simulink model "Tx_sim"  (R2021b)
settings: Solver=VariableStepAuto  StartTime=0.0  StopTime=10.0  RelTol=1e-3
settings Model: Creator=Blade  LastModifiedBy=Blade

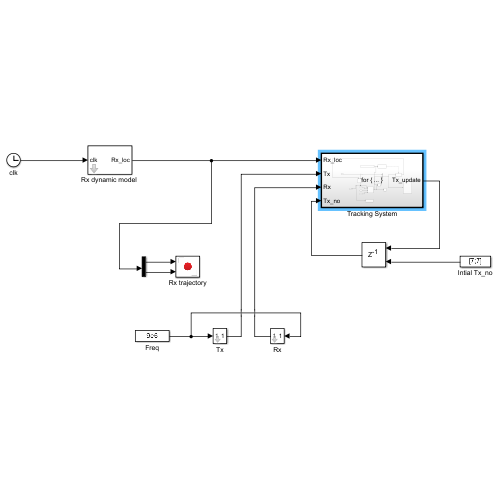
[thumbnail: Simulink's stored preview of the top-level diagram]
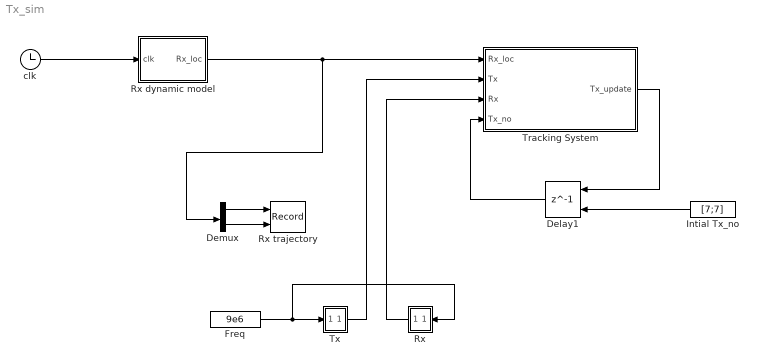
== system Tx_sim ==
  Delay1 : Delay  DelayLength=1  InitialConditionSource=Input port  InitialCondition=[2,2]
      settings: InputPortMap=u0,p4
  Demux : Demux  Outputs=2
  Freq : Constant  Value=9e6
  Intial Tx_no : Constant  Value=[7;7]  VectorParams1D=off
  Rx : Subsystem  mask{dout=1/3*100e-3, phi=0.15, s=800e-6, w=1200e-6, CP=0, SR=0.01}
      mask prompts: dout "out diameter"; phi "fillfact"; s "track spacing"; w "track width"; CP "parasitic capacitance"; SR "source resistance"
      mask TypeOptions dout: Constant1/Value
      mask TypeOptions phi: Constant2/Value
      mask TypeOptions s: Constant3/Value
      mask TypeOptions w: Constant4/Value
      mask TypeOptions CP: Constant6/Value
      mask TypeOptions SR: Constant7/Value
  "Rx dynamic model " : Subsystem  mask{initx=1/2*100e-3*(7+1), inity=1/2*100e-3*(7+1), v_min=[0.01,0.01], v_max=[0.01,0.01]}
      mask prompts: initx "Rx initial x"; inity "Rx initial y"; v_min "Rx min speed"; v_max "Rx max speed"
      mask TypeOptions initx: Delay1/InitialCondition
      mask TypeOptions inity: Delay2/InitialCondition
      mask TypeOptions v_min: Constant/Value
      mask TypeOptions v_max: Constant1/Value
  Rx trajectory : Record  FileSettingsInternal="{\"entries\":[{\"content\":{\"excelSettings\":{\"content\":{},\"type\":\"Streamout.ExcelSettings\"}},\"type\":\"Streamout.FileSettingStorage\",\"uuid\":\"5ea7622f-e3f2-434e-8594-dca06b2b01b1\"}],\"packageUris\":[\"http://schema.mathworks.com/mf0/streamout_blocks/R2020a\"],\"version\":\"1.0\"}"  Layout=[1 1]  SignalsInternal="{\"entries\":[{\"content\":{\"signals\":[{\"content\":{\"blockPath\":[\"untitled/Rx trajectory\"],\"channel\":[],\"dimensions\":[1],\"domain\":\"untitled/Rx trajectory\",\"lineColor\":\"#22b573\",\"plots\":[],\"port\":1,\"sid\":[\"\"],\"signalID\":1150986,\"signalName\":\"Demux:1\"},\"type\":\"RecordBlkView.Signal\",\"uuid\":\"ce63fc5f-71f3-4bbf-96f5-20283097e031\"},{\"content\":{\"blockPath\":[\"untitled/Rx trajectory\"],\"channel\":[],\"dimensions\":[1],\"domain\":\"untitled/Rx trajectory\",\"lineColor\":\"#0072bd\",\"plots\":[],\"port\":2,\"sid\":[\"\"],\"signalID\":1150990,\"signalName\":\"Demux:2\"},\"type\":\"RecordBlkView.Signal\",\"uuid\":\"feeefa71-ac5c-4467-a179-d29ba9ae9525\"}]},\"type\":\"RecordBlkView.InputSignals\",\"uuid\":\"cc4d89dd-a1d8-473b-8fe9-6d08d22a2a17\"}],\"packageUris\":[\"http://schema.mathworks.com/mf0/streamout_blocks/R2020a\"],\"version\":\"1.0\"}"  VisualizationBindings="{\"xyplotplugin\":{\"info\":[{\"series\":[],\"subplotID\":1}]}}"  CompatibilityTag=XY
  Tracking System : Subsystem  TreatAsAtomicUnit=on
  Tx : Subsystem  mask{dout=100e-3, phi=0.25, s=3*2500e-6, w=2500e-6, CP=0, SR=0.01}
      mask prompts: dout "out diameter"; phi "fillfact"; s "track spacing"; w "track width"; CP "parasitic capacitance"; SR "source resistance"
      mask TypeOptions dout: Constant1/Value
      mask TypeOptions phi: Constant2/Value
      mask TypeOptions s: Constant3/Value
      mask TypeOptions w: Constant4/Value
      mask TypeOptions CP: Constant6/Value
      mask TypeOptions SR: Constant7/Value
  clk : Clock
  wires:
  Tracking System/1(Tx_update) -> Delay1/1
  Tx/1(Out1) -> Tracking System/2(Tx)
  clk/1 -> "Rx dynamic model "/1(clk)
  Demux/1 -> Rx trajectory/1
  Delay1/1 -> Tracking System/4(Tx_no)
  Demux/2 -> Rx trajectory/2
  Rx/1(Out1) -> Tracking System/3(Rx)
  Freq/1 -> Rx/1(In1), Tx/1(In1)
  "Rx dynamic model "/1(Rx_loc) -> Demux/1, Tracking System/1(Rx_loc)
  Intial Tx_no/1 -> Delay1/2

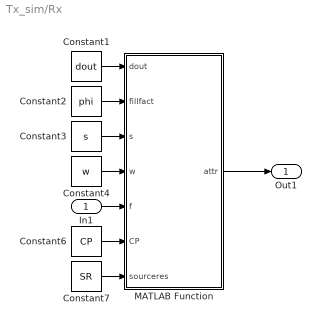
== system Tx_sim/Rx ==
  In1 : Inport
  Constant1 : Constant  Value=dout
  Constant2 : Constant  Value=phi
  Constant3 : Constant  Value=s
  Constant4 : Constant  Value=w
  Constant6 : Constant  Value=CP
  Constant7 : Constant  Value=SR
  MATLAB Function : MATLAB Function  TreatAsAtomicUnit=on
  Out1 : Outport
  wires:
  MATLAB Function/1(attr) -> Out1/1
  Constant7/1 -> MATLAB Function/7(sourceres)
  Constant1/1 -> MATLAB Function/1(dout)
  Constant2/1 -> MATLAB Function/2(fillfact)
  Constant3/1 -> MATLAB Function/3(s)
  Constant4/1 -> MATLAB Function/4(w)
  In1/1 -> MATLAB Function/5(f)
  Constant6/1 -> MATLAB Function/6(CP)

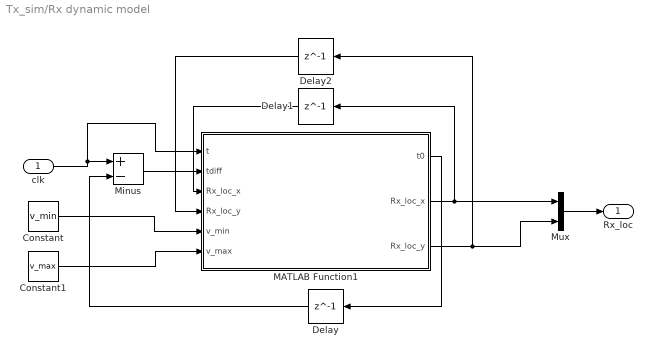
== system Tx_sim/Rx dynamic model  ==
  clk : Inport
  Constant : Constant  Value=v_min  VectorParams1D=off
  Constant1 : Constant  Value=v_max  VectorParams1D=off
  Delay : Delay  DelayLength=1  InitialCondition=0
  Delay1 : Delay  DelayLength=1  InitialCondition=initx
  Delay2 : Delay  DelayLength=1  InitialCondition=inity
  MATLAB Function1 : MATLAB Function  TreatAsAtomicUnit=on
  Minus : Sum  Inputs=+-
  Mux : Mux  Inputs=2
  Rx_loc : Outport
  wires:
  MATLAB Function1/3(Rx_loc_y) -> Delay2/1, Mux/2
  Delay/1 -> Minus/2
  clk/1 -> MATLAB Function1/1(t), Minus/1
  Delay2/1 -> MATLAB Function1/4("Rx_loc_y ")
  MATLAB Function1/1(t0) -> Delay/1
  Minus/1 -> MATLAB Function1/2(tdiff)
  Delay1/1 -> MATLAB Function1/3("Rx_loc_x ")
  MATLAB Function1/2(Rx_loc_x) -> Delay1/1, Mux/1
  Mux/1 -> Rx_loc/1
  Constant/1 -> MATLAB Function1/5(v_min)
  Constant1/1 -> MATLAB Function1/6(v_max)

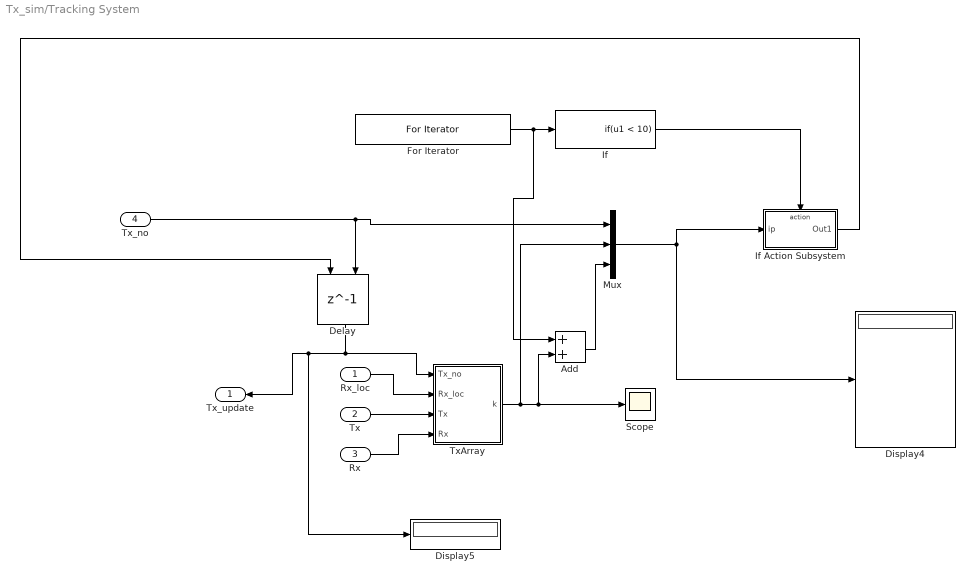
== system Tx_sim/Tracking System ==
  Rx_loc : Inport
  Tx : Inport  Port=2
  Rx : Inport  Port=3
  Tx_no : Inport  Port=4
  Add : Sum
  Delay : Delay  DelayLength=1  InitialConditionSource=Input port  InitialCondition=0
      settings: InputPortMap=u0,p4
  Display4 : Display
  Display5 : Display
  For Iterator : ForIterator  ResetStates=reset  IterationLimit=10  IterationVariableDataType=double
  If : If  IfExpression=u1 < 10  ShowElse=off
  If Action Subsystem : Subsystem  TreatAsAtomicUnit=on
  Mux : Mux  Inputs=3
  Scope : Scope
  TxArray : Subsystem
  Tx_update : Outport
  wires:
  Rx/1 -> TxArray/4(Rx)
  Tx/1 -> TxArray/3(Tx)
  Rx_loc/1 -> TxArray/2(Rx_loc)
  TxArray/1(k) -> Mux/2, Scope/1, Add/2
  Tx_no/1 -> Delay/2, Mux/1
  Delay/1 -> TxArray/1(Tx_no), Display5/1, Tx_update/1
  Mux/1 -> If Action Subsystem/1("ip "), Display4/1
  For Iterator/1 -> Add/1, If/1
  If/1 -> If Action Subsystem/Action
  Add/1 -> Mux/3
  If Action Subsystem/1(Out1) -> Delay/1

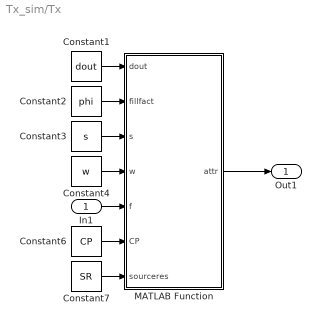
== system Tx_sim/Tx ==
  In1 : Inport
  Constant1 : Constant  Value=dout
  Constant2 : Constant  Value=phi
  Constant3 : Constant  Value=s
  Constant4 : Constant  Value=w
  Constant6 : Constant  Value=CP
  Constant7 : Constant  Value=SR
  MATLAB Function : MATLAB Function  TreatAsAtomicUnit=on
  Out1 : Outport
  wires:
  MATLAB Function/1(attr) -> Out1/1
  Constant7/1 -> MATLAB Function/7(sourceres)
  Constant1/1 -> MATLAB Function/1(dout)
  Constant2/1 -> MATLAB Function/2(fillfact)
  Constant3/1 -> MATLAB Function/3(s)
  Constant4/1 -> MATLAB Function/4(w)
  In1/1 -> MATLAB Function/5(f)
  Constant6/1 -> MATLAB Function/6(CP)

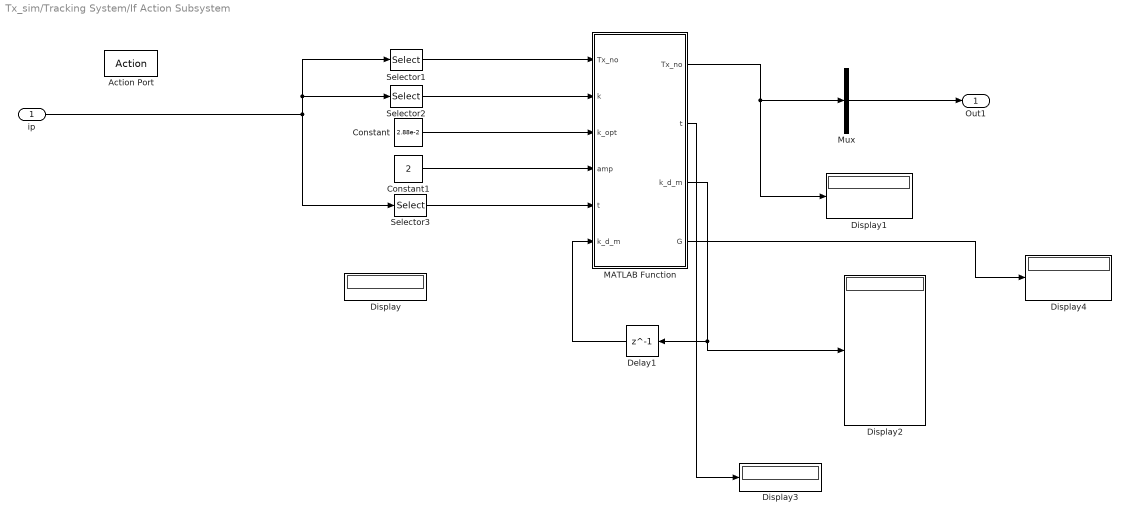
== system Tx_sim/Tracking System/If Action Subsystem ==
  "ip " : Inport
  Action Port : ActionPort  ActionPortLabel=if(u1 < 10)
  Constant : Constant  Value=2.88e-2
  Constant1 : Constant  Value=2
  Delay1 : Delay  DelayLength=1  InitialCondition=zeros(1,9)
  Display{,1..4} (5 alike) : Display
  MATLAB Function : MATLAB Function  TreatAsAtomicUnit=on
  Mux : Mux  Inputs=1
  Selector1 : Selector  InputPortWidth=4  IndexOptions=Index vector (dialog)  Indices=[1;2]  OutputSizes=1
  Selector2 : Selector  InputPortWidth=4  IndexOptions=Index vector (dialog)  Indices=3  OutputSizes=1
  Selector3 : Selector  InputPortWidth=4  IndexOptions=Index vector (dialog)  Indices=4  OutputSizes=1
  Out1 : Outport
  wires:
  MATLAB Function/2(t) -> Display3/1
  "ip "/1 -> Selector2/1, Selector1/1, Selector3/1
  MATLAB Function/3(k_d_m) -> Display2/1, Delay1/1
  Constant/1 -> MATLAB Function/3(k_opt)
  Delay1/1 -> MATLAB Function/6("k_d_m ")
  MATLAB Function/1(Tx_no) -> Display1/1, Mux/1
  Selector1/1 -> MATLAB Function/1("Tx_no ")
  Selector2/1 -> MATLAB Function/2(k)
  Constant1/1 -> MATLAB Function/4(amp)
  Selector3/1 -> MATLAB Function/5("t ")
  MATLAB Function/4(G) -> Display4/1
  Mux/1 -> Out1/1

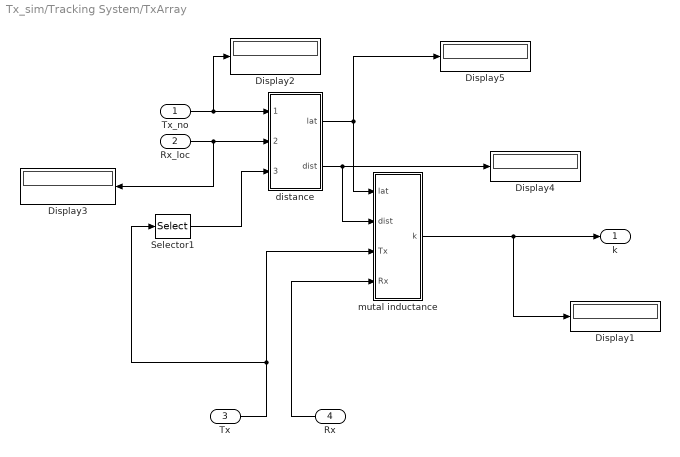
== system Tx_sim/Tracking System/TxArray ==
  Tx_no : Inport
  Rx_loc : Inport  Port=2
  Tx : Inport  Port=3
  Rx : Inport  Port=4
  " mutal inductance" : Subsystem
  Display{1..5} (5 alike) : Display
  Selector1 : Selector  InputPortWidth=14  IndexOptions=Index vector (dialog)  Indices=1  OutputSizes=1
  distance : Subsystem
  k : Outport
  wires:
  Tx/1 -> Selector1/1, " mutal inductance"/3(Tx)
  distance/1(lat) -> " mutal inductance"/1(lat), Display5/1
  Rx/1 -> " mutal inductance"/4(Rx)
  Tx_no/1 -> Display2/1, distance/1(Tx_no)
  Rx_loc/1 -> Display3/1, distance/2(Rx_loc)
  Selector1/1 -> distance/3(Tx_dia)
  " mutal inductance"/1(k) -> Display1/1, k/1
  distance/2(dist) -> " mutal inductance"/2(dist), Display4/1

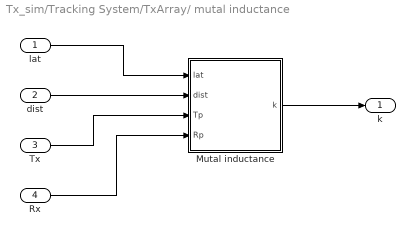
== system Tx_sim/Tracking System/TxArray/ mutal inductance ==
  lat : Inport
  dist : Inport  Port=2
  Tx : Inport  Port=3
  Rx : Inport  Port=4
  Mutal inductance : MATLAB Function  TreatAsAtomicUnit=on
  k : Outport
  wires:
  lat/1 -> Mutal inductance/1(lat)
  dist/1 -> Mutal inductance/2(dist)
  Tx/1 -> Mutal inductance/3(Tp)
  Rx/1 -> Mutal inductance/4(Rp)
  Mutal inductance/1(k) -> k/1

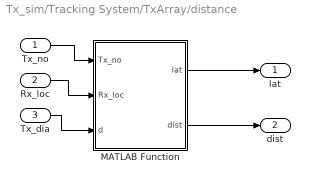
== system Tx_sim/Tracking System/TxArray/distance ==
  Tx_no : Inport
  Rx_loc : Inport  Port=2
  Tx_dia : Inport  Port=3
  MATLAB Function : MATLAB Function  TreatAsAtomicUnit=on
  lat : Outport
  dist : Outport  Port=2
  wires:
  Tx_dia/1 -> MATLAB Function/3(d)
  Tx_no/1 -> MATLAB Function/1(Tx_no)
  Rx_loc/1 -> MATLAB Function/2(Rx_loc)
  MATLAB Function/1(lat) -> lat/1
  MATLAB Function/2(dist) -> dist/1

== matlab function Tx_sim/Tracking System/TxArray/distance/MATLAB Function ==
  data: Tx_no input; Rx_loc input; d input; lat output; dist output
function [lat, dist] = distance(Tx_no, Rx_loc, d)

coder.extrinsic('lat_dist');
coder.extrinsic('vertical_dist');


lat = 0;
dist = 0;

lat = lat_dist(Tx_no, Rx_loc,d);
dist = vertical_dist(Tx_no);
dist = dist + 5e-2;
end

== matlab function Tx_sim/Tracking System/TxArray/ mutal inductance/Mutal inductance ==
  data: lat input; dist input; Tp input; Rp input; k output
function  k = solenoid_MI(lat,dist,Tp,Rp)


coder.extrinsic('MI');

% M = 0;
k = 0;

[~,k] = MI(lat,dist,Tp,Rp);

if k < 0
    k = 0;
end

end

== matlab function Tx_sim/Tx/MATLAB Function ==
  data: dout input; attr output; fillfact input; s input; w input; f input; CP input; sourceres input
function attr = PCBPhySim(dout,fillfact,s,w,f,CP,sourceres)


y = PCBCoil(dout,fillfact,s,w,f,CP,'square',sourceres);

attr = [y.dout,
    y.din,
    y.fillfact,
    y.w,
    y.s,
    y.n,
    y.L,
    y.Rs,
    y.Q,
    y.C,
    y.CP,
    y.coilZ,
    y.fSRF
    y.f];

== matlab function Tx_sim/Tracking System/If Action Subsystem/MATLAB Function ==
  data: Tx_no input; k input; Tx_no output; k_opt input; amp input; t input; t output; k_d_m output; k_d_m input; G output
function [Tx_no,t,k_d_m,G] = Controller(Tx_no, k,k_opt,amp,t,k_d_m)

t = round(t);
k_diff = abs(k_opt-k)/k_opt;

k_d_m (t) = k_diff;
    
G = round(amp*k_d_m(1));

if t < 9
    dir_att = [-1,-1; -1,0; 0,-1; 1,1; 1,0; 0,1; 1,-1; -1,1];
    
    

    Tx_no =G*dir_att(t,:)'+Tx_no;
    
    
    

else
    
    dir_cand = [0,0; -1,-1; -1,0; 0,-1; 1,1; 1,0; 0,1; 1,-1; -1,1]; 
    [~, index] = min(k_d_m);
    dir_opt = dir_cand(index,:);
    G = round(amp*k_d_m(1));
    Tx_no = Tx_no+ dir_opt'*G;

   
end

== matlab function Tx_sim/Rx/MATLAB Function ==
  data: dout input; attr output; fillfact input; s input; w input; f input; CP input; sourceres input
function attr = PCBPhySim(dout,fillfact,s,w,f,CP,sourceres)


y = PCBCoil(dout,fillfact,s,w,f,CP,'square',sourceres);

attr = [y.dout,
    y.din,
    y.fillfact,
    y.w,
    y.s,
    y.n,
    y.L,
    y.Rs,
    y.Q,
    y.C,
    y.CP,
    y.coilZ,
    y.fSRF
    y.f];

== matlab function Tx_sim/Rx dynamic model /MATLAB Function1 ==
  data: t input; tdiff input; t0 output; Rx_loc_x output; Rx_loc_x input; Rx_loc_y input; Rx_loc_y output; v_min input; v_max input
function [t0, Rx_loc_x, Rx_loc_y] = dynamic_on_TxArray(t, tdiff, Rx_loc_x, Rx_loc_y, v_min, v_max)
% if t>=0 && t < 8
%     tdiff = 0;
% elseif t>=10 && t < 19
%     tdiff = 0;
% elseif t>=20 && t < 29
%     tdiff = 0;
% elseif t>=30 && t < 39
%     tdiff = 0;   
% elseif t>=40 && t < 49
%     tdiff = 0;
% elseif t>=50 && t < 59
%     tdiff = 0;
% elseif t>=60 && t < 69
%     tdiff = 0;
% elseif t>=70 && t < 79
%     tdiff = 0;
% elseif t>=80 && t < 89
%     tdiff = 0;
% elseif t>=90 && t < 99
%     tdiff = 0;
% end

d = 0;
Rx_loc = [Rx_loc_x,Rx_loc_y];
coder.extrinsic('dynamic');
Rx_loc = dynamic(tdiff,Rx_loc,v_min,v_max);
Rx_loc_x = 0;
Rx_loc_y = 0;
Rx_loc_x = Rx_loc(1);
Rx_loc_y = Rx_loc(2);

t0 = t;
